simulink model "Dyn_6DoF_v2_0_r2019b"  (R2019b)
settings: Solver=ode4  StartTime=0.0  StopTime=simInit.TSIM  FixedStep=simInit.dt  MaxStep=simInit.dt  RelTol=1e-3
InitFcn:
  | close all
undefined symbols (not defined in the file): __PRM__SERIALIZED__DATA__, act, constr, DE2019, DiscIntNeverNeededParam, ENVMT, omega_rate_max, params, simInit, SubsystemReferenceBlock
libraries: simulink x16, simulink_extras x3
(part 1 of 3)
Description:
  | % Copyright 2020 Delft University of Technology
  | %
  | % Licensed under the Apache License, Version 2.0 (the "License");
  | % you may not use this file except in compliance with the License.
  | % You may obtain a copy of the License at
  | %
  | %      http://www.apache.org/licenses/LICENSE-2.0
  | %
  | % Unless required by applicable law or agreed to in writing, software
  | % distributed under the License is distributed on an "AS IS" BASIS,
  | % WITHOUT WARRANTIES OR CONDITIONS OF ANY KIND, either express or implied.
  | % See the License for the specific language governing permissions and
  | % limitations under the License.
settings Model: SimulationMode=accelerator  NumberOfSteps=50  ExtModeTrigDuration=100  Creator=Sebastian  LastModifiedBy=dylaneijkelhof
settings SolverCC: SolverJacobianMethodControl=FullAnalytical
settings DataIOCC: InitialState=testPoint  SaveFormat=Structure  SignalLogging=off  DSMLogging=off  SaveTime=off  ReturnWorkspaceOutputs=off  StateSaveName=tmp_raccel_xout  SignalLoggingName=logged_signals  LoggingFileName=log
settings OptimizationCC: BlockReduction=off  EfficientMapNaN2IntZero=off  LifeSpan=inf
settings DebuggingCC: ArtificialAlgebraicLoopMsg=none  SaveWithDisabledLinksMsg=none  SaveWithParameterizedLinksMsg=none  MaskedZcDiagnostic=none  IgnoredZcDiagnostic=none  InheritedTsInSrcMsg=none  TasksWithSamePriorityMsg=none  SigSpecEnsureSampleTimeMsg=none  ParameterPrecisionLossMsg=none  UnconnectedInputMsg=none  UnconnectedOutputMsg=none  UnconnectedLineMsg=none  BusObjectLabelMismatch=none  RootOutportRequireBusObject=none  UnknownTsInhSupMsg=none  ModelReferenceDataLoggingMessage=none  ModelReferenceSymbolNameMessage=none  InitInArrayFormatMsg=none  SFUnusedDataAndEventsDiag=none  SFUnexpectedBacktrackingDiag=none  SFInvalidInputDataAccessInChartInitDiag=none  SFNoUnconditionalDefaultTransitionDiag=none  SFTransitionOutsideNaturalParentDiag=none  SFUnreachableExecutionPathDiag=none  SFUndirectedBroadcastEventsDiag=none  SFTransitionActionBeforeConditionDiag=none  SFTemporalDelaySmallerThanSampleTimeDiag=none  SFSelfTransitionDiag=none  SFExecutionAtInitializationDiag=none  SFMachineParentedDataDiag=none  UnitsInconsistencyMsg=none  ArithmeticOperatorsInVariantConditions=warning
settings HardwareCC: ProdBitPerLong=64  ProdLongLongMode=on  ProdHWDeviceType=Custom Processor->Custom Processor  TargetBitPerLong=64  TargetBitPerPointer=64  TargetBitPerSizeT=64  TargetBitPerPtrDiffT=64  TargetLargestAtomicFloat=Float  TargetLongLongMode=on  TargetIntDivRoundTo=Zero  TargetEndianess=LittleEndian  TargetWordSize=64  TargetHWDeviceType=Custom Processor->MATLAB Host Computer
settings ModelReferenceCC: PropagateSignalLabelsOutOfModel=off
settings SFSimCC: SimUseLocalCustomCode=off  CustomCodeUndefinedFunction=UseInterfaceOnly
settings CodeAppCC: MaxIdLength=128
settings GRTTargetCC: TargetLangStandard=C89/C90 (ANSI)  CombineOutputUpdateFcns=off  GRTInterface=on
settings ConfigComp: CovMetricSettings=dw  CovHtmlReporting=on  CovSaveCumulativeToWorkspaceVar=on  CovSaveSingleToWorkspaceVar=on  CovExternalEMLEnable=off
settings SimscapeCC: SimscapeNormalizeSystem=off
settings ConfigurationSet: Description=SimMechanics 2G

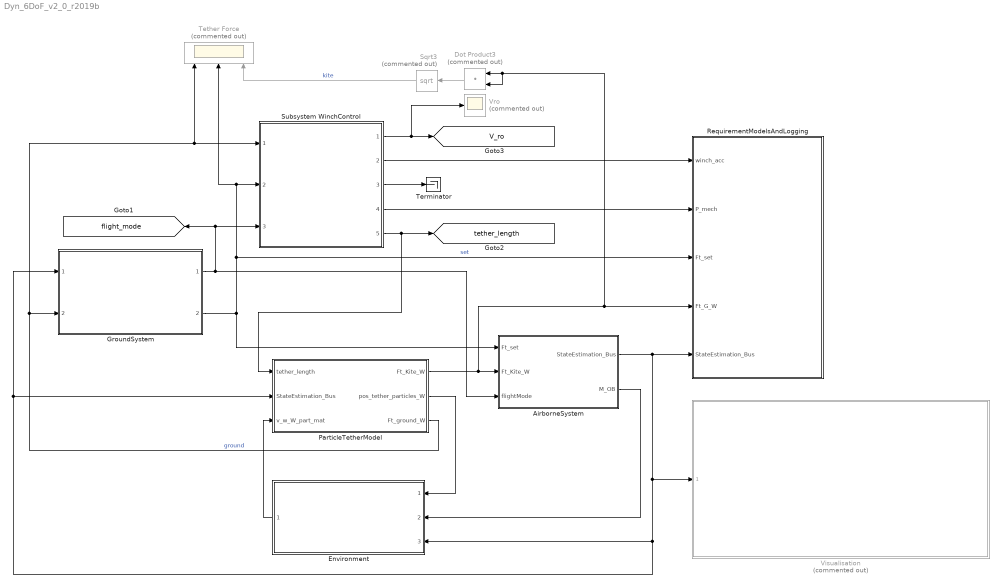
== system Dyn_6DoF_v2_0_r2019b ==
  AirborneSystem : Subsystem
  Dot Product3 : DotProduct  Commented=on  InputSameDT=on  OutDataTypeStr=Inherit: Inherit via internal rule
  Environment : Subsystem  BlockKeywords=__PRM__SERIALIZED__DATA__:SubsystemReferenceBlock  ReferencedSubsystem=Environment
  GroundSystem : Subsystem  BlockKeywords=__PRM__SERIALIZED__DATA__:SubsystemReferenceBlock  ReferencedSubsystem=GroundSystem
  ParticleTetherModel : Subsystem
  RequirementModelsAndLogging : Subsystem  mask{log_sample_time=0.2}
  Sqrt3 : Sqrt  Commented=on  SaturateOnIntegerOverflow=on
  Subsystem WinchControl : Subsystem  BlockKeywords=__PRM__SERIALIZED__DATA__:SubsystemReferenceBlock  ReferencedSubsystem=WinchControl
  Terminator : Terminator
  Tether Force : Scope  Commented=on  NumInputPorts=3
  Visualisation : Subsystem  Commented=on  ReferencedSubsystem=Visualisation
  Vro : Scope  Commented=on
  tag scope: V_ro=global, flight_mode=global, tether_length=global
  wires:
  GroundSystem/1 -> AirborneSystem/3(flightMode), Subsystem WinchControl/3, [flight_mode]
  GroundSystem/2 -> Subsystem WinchControl/2, Tether Force/2, RequirementModelsAndLogging/3(Ft_set), AirborneSystem/1(Ft_set)  "set"
  AirborneSystem/2(M_OB) -> Environment/2
  AirborneSystem/1(StateEstimation_Bus) -> RequirementModelsAndLogging/5(StateEstimation_Bus), Environment/3, GroundSystem/1, ParticleTetherModel/2(StateEstimation_Bus), Visualisation/1
  ParticleTetherModel/2(pos_tether_particles_W) -> Environment/1
  Environment/1 -> ParticleTetherModel/3(v_w_W_part_mat)
  Subsystem WinchControl/1 -> Vro/1, [V_ro]
  ParticleTetherModel/3(Ft_ground_W) -> GroundSystem/2, Subsystem WinchControl/1, Tether Force/1  "ground"
  Subsystem WinchControl/3 -> Terminator/1
  Subsystem WinchControl/2 -> RequirementModelsAndLogging/1(winch_acc)
  Subsystem WinchControl/4 -> RequirementModelsAndLogging/2(P_mech)
  Subsystem WinchControl/5 -> [tether_length], ParticleTetherModel/1(tether_length)
  Sqrt3/1 -> Tether Force/3  "kite"
  Dot Product3/1 -> Sqrt3/1
  ParticleTetherModel/1(Ft_Kite_W) -> RequirementModelsAndLogging/4(Ft_G_W), Dot Product3/2, Dot Product3/1, AirborneSystem/2(Ft_Kite_W)

== system Dyn_6DoF_v2_0_r2019b/AirborneSystem ==
  Ft_set : Inport
  Ft_Kite_W : Inport  Port=2
  flightMode : Inport  Port=3
  6DoFDynamics : Subsystem
  Dot Product : DotProduct  InputSameDT=on  OutDataTypeStr=Inherit: Inherit via internal rule
  FlightControlSystem : Subsystem
  ForcesAndTorques : Subsystem
  Sqrt : Sqrt  SaturateOnIntegerOverflow=on
  StateEstimation_Bus : Outport  VectorParamsAs1DForOutWhenUnconnected=off
  M_OB : Outport  Port=2  VectorParamsAs1DForOutWhenUnconnected=off
  wires:
  6DoFDynamics/2(StateEstimation_Bus) -> FlightControlSystem/4(StateEstimation_Bus), ForcesAndTorques/3(StateEstimation_Bus), StateEstimation_Bus/1  "StateEstimation_Bus"
  6DoFDynamics/1(M_OB) -> M_OB/1
  Ft_Kite_W/1 -> 6DoFDynamics/1(F_t_W), Dot Product/2, Dot Product/1
  Dot Product/1 -> Sqrt/1
  Ft_set/1 -> FlightControlSystem/2(Ft_set)
  Sqrt/1 -> FlightControlSystem/3(Ft_tot_kite)
  ForcesAndTorques/1(F_a_B) -> 6DoFDynamics/2(F_a_B), FlightControlSystem/1(F_a_B)
  FlightControlSystem/2(throttle/brake) -> ForcesAndTorques/2(throttle/brake)
  ForcesAndTorques/2(F_p_B) -> 6DoFDynamics/3(F_p_B)
  ForcesAndTorques/3(M_a_B) -> 6DoFDynamics/4(Torques), FlightControlSystem/5(M_a_B)
  FlightControlSystem/1(u_controlsurfaces) -> ForcesAndTorques/1(u_cmd)
  flightMode/1 -> FlightControlSystem/6(fm)

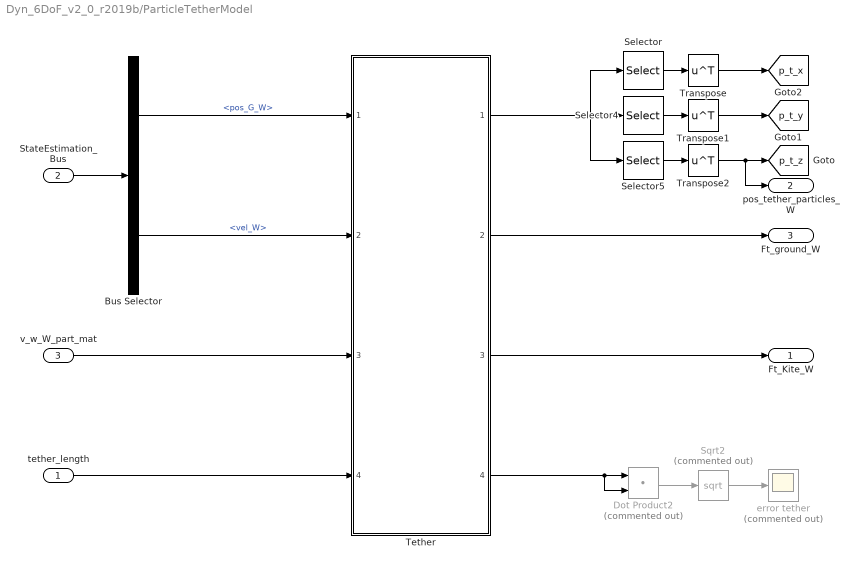
== system Dyn_6DoF_v2_0_r2019b/ParticleTetherModel ==
  tether_length : Inport
  StateEstimation_Bus : Inport  Port=2
  v_w_W_part_mat : Inport  Port=3
  Bus Selector : BusSelector  OutputSignals=pos_G_W,vel_W
  Dot Product2 : DotProduct  Commented=on  InputSameDT=on  OutDataTypeStr=Inherit: Inherit via internal rule
  Selector : Selector  NumberOfDimensions=2  InputPortWidth=3  IndexOptions=Index vector (dialog),Select all  Indices=1,1  OutputSizes=1,1
  Selector4 : Selector  NumberOfDimensions=2  InputPortWidth=3  IndexOptions=Index vector (dialog),Select all  Indices=2,1  OutputSizes=1,1
  Selector5 : Selector  NumberOfDimensions=2  InputPortWidth=3  IndexOptions=Index vector (dialog),Select all  Indices=3,1  OutputSizes=1,1
  Sqrt2 : Sqrt  Commented=on  SaturateOnIntegerOverflow=on
  Tether : Subsystem  ReferencedSubsystem=Tether_dynamics_R2019B
  Transpose : Math  Operator=transpose  SignedPower=off  SaturateOnIntegerOverflow=on
  Transpose1 : Math  Operator=transpose  SignedPower=off  SaturateOnIntegerOverflow=on
  Transpose2 : Math  Operator=transpose  SignedPower=off  SaturateOnIntegerOverflow=on
  error tether : Scope  Commented=on
  Ft_Kite_W : Outport  VectorParamsAs1DForOutWhenUnconnected=off
  pos_tether_particles_W : Outport  Port=2  VectorParamsAs1DForOutWhenUnconnected=off
  Ft_ground_W : Outport  Port=3  VectorParamsAs1DForOutWhenUnconnected=off
  tag scope: p_t_x=global, p_t_y=global, p_t_z=global
  wires:
  v_w_W_part_mat/1 -> Tether/3
  StateEstimation_Bus/1 -> Bus Selector/1
  Bus Selector/1 -> Tether/1  "<pos_G_W>"
  Bus Selector/2 -> Tether/2  "<vel_W>"
  Selector4/1 -> Transpose1/1
  Selector5/1 -> Transpose2/1
  Selector/1 -> Transpose/1
  Transpose/1 -> [p_t_x]
  Transpose1/1 -> [p_t_y]
  Transpose2/1 -> pos_tether_particles_W/1, [p_t_z]
  Tether/4 -> Dot Product2/2, Dot Product2/1
  Tether/1 -> Selector/1, Selector5/1, Selector4/1
  Dot Product2/1 -> Sqrt2/1
  Sqrt2/1 -> error tether/1
  Tether/2 -> Ft_ground_W/1
  Tether/3 -> Ft_Kite_W/1
  tether_length/1 -> Tether/4

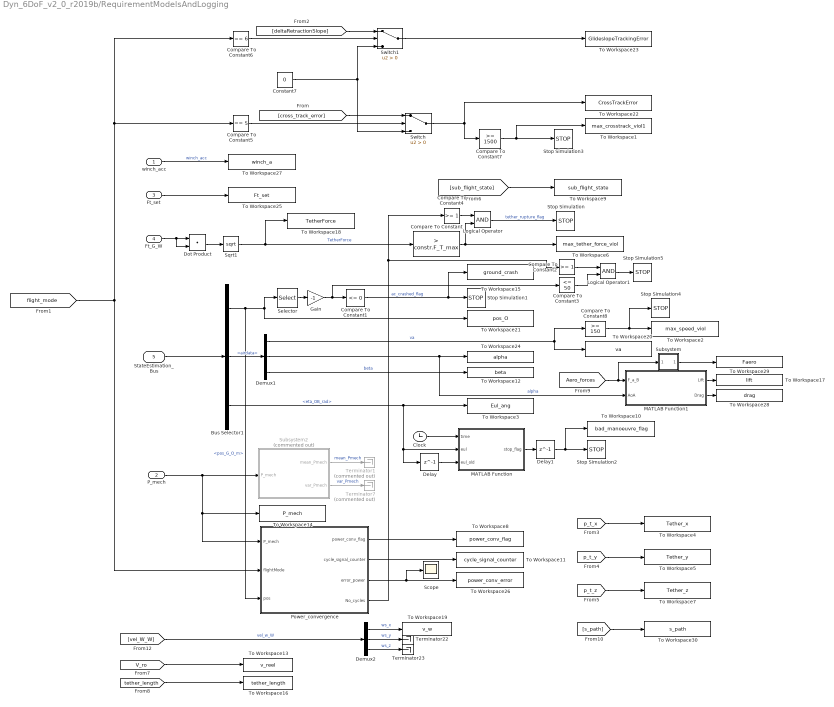
== system Dyn_6DoF_v2_0_r2019b/RequirementModelsAndLogging ==
  winch_acc : Inport
  P_mech : Inport  Port=2
  Ft_set : Inport  Port=3
  Ft_G_W : Inport  Port=4
  StateEstimation_Bus : Inport  Port=5
  Bus Selector1 : BusSelector  OutputSignals=pos_G_O_m,airdata,eta_OB_rad
  Clock : Clock
  Compare To Constant : simulink/Logic and Bit Operations/Compare To Constant  relop=>  const=constr.F_T_max  OutDataTypeStr=boolean
  Compare To Constant1 : simulink/Logic and Bit Operations/Compare To Constant  relop=<=  const=0  OutDataTypeStr=boolean
  Compare To Constant2 : simulink/Logic and Bit Operations/Compare To Constant  relop=>=  const=1  OutDataTypeStr=boolean
  Compare To Constant3 : simulink/Logic and Bit Operations/Compare To Constant  relop=<=  const=50  OutDataTypeStr=boolean
  Compare To Constant4 : simulink/Logic and Bit Operations/Compare To Constant  relop=>=  const=1  OutDataTypeStr=boolean
  Compare To Constant5 : simulink/Logic and Bit Operations/Compare To Constant  relop===  const=5  OutDataTypeStr=boolean
  Compare To Constant6 : simulink/Logic and Bit Operations/Compare To Constant  relop===  const=6  OutDataTypeStr=boolean
  Compare To Constant7 : simulink/Logic and Bit Operations/Compare To Constant  relop=>=  const=1500  OutDataTypeStr=boolean
  Compare To Constant8 : simulink/Logic and Bit Operations/Compare To Constant  relop=>=  const=150  OutDataTypeStr=boolean
  Constant7 : Constant  Value=0
  Delay : Delay  DelayLength=1  InitialCondition=zeros(3,1)
  Delay1 : Delay  DelayLength=1
  Demux1 : Demux  Outputs=3
  Demux2 : Demux  Outputs=3
  Dot Product : DotProduct  InputSameDT=on  OutDataTypeStr=Inherit: Inherit via internal rule
  Gain : Gain  Gain=-1
  Logical Operator : Logic  AllPortsSameDT=off  OutDataTypeStr=boolean
  Logical Operator1 : Logic  AllPortsSameDT=off  OutDataTypeStr=boolean
  MATLAB Function : MATLAB Function  TreatAsAtomicUnit=on
  MATLAB Function1 : MATLAB Function  TreatAsAtomicUnit=on
  Power_convergence : Subsystem  mask{sample_time=simInit.Ts_power_conv_check, threshold=130000, min_cycles=3, pos_threshold=400}
      mask prompts: threshold "start_threshold"; min_cycles "minimum_cycles"; pos_threshold "maximum position distance"
  Scope : Scope
  Selector : Selector  InputPortWidth=3  IndexOptions=Index vector (dialog)  Indices=3  OutputSizes=1
  Sqrt1 : Sqrt  SaturateOnIntegerOverflow=on
  Stop Simulation{,1..5} (6 alike) : Stop
  Subsystem : Subsystem
      mask Display: disp('norm()')
  Subsystem2 : Subsystem  Commented=on
  Switch : Switch  Criteria=u2 > Threshold
  Switch1 : Switch  Criteria=u2 > Threshold
  Terminator1 : Terminator  Commented=on
  Terminator22 : Terminator
  Terminator23 : Terminator
  Terminator7 : Terminator  Commented=on
  To Workspace1 : ToWorkspace  VariableName=max_crosstrack_viol1  SampleTime=-1
      settings: MaxDataPoints=1
  To Workspace10 : ToWorkspace  VariableName=bad_manoeuvre_flag  SampleTime=-1
      settings: MaxDataPoints=1
  To Workspace11 : ToWorkspace  VariableName=cycle_signal_counter  SaveFormat=Timeseries  SampleTime=-1
      settings: MaxDataPoints=1  Save2DSignal=2-D array (concatenate along first dimension)
  To Workspace12 : ToWorkspace  VariableName=beta  SaveFormat=Timeseries  SampleTime=simInit.AttLoggingTs
      settings: Save2DSignal=2-D array (concatenate along first dimension)
  To Workspace13 : ToWorkspace  VariableName=v_reel  SaveFormat=Timeseries  SampleTime=simInit.PLoggingTs
  To Workspace14 : ToWorkspace  VariableName=P_mech  SaveFormat=Timeseries  SampleTime=simInit.PLoggingTs
  To Workspace15 : ToWorkspace  VariableName=ground_crash  SampleTime=-1
      settings: MaxDataPoints=1
  To Workspace16 : ToWorkspace  VariableName=tether_length  SaveFormat=Timeseries  SampleTime=simInit.AttLoggingTs
  To Workspace17 : ToWorkspace  VariableName=lift  SaveFormat=Timeseries  SampleTime=simInit.AttLoggingTs
      settings: Save2DSignal=2-D array (concatenate along first dimension)
  To Workspace18 : ToWorkspace  VariableName=TetherForce  SaveFormat=Timeseries  SampleTime=simInit.FtLoggingTs
  To Workspace19 : ToWorkspace  VariableName=v_w  SaveFormat=Timeseries  SampleTime=simInit.PLoggingTs
  To Workspace2 : ToWorkspace  VariableName=max_speed_viol  SampleTime=-1
      settings: MaxDataPoints=1
  To Workspace20 : ToWorkspace  VariableName=va  SaveFormat=Timeseries  SampleTime=simInit.AttLoggingTs
      settings: Save2DSignal=2-D array (concatenate along first dimension)
  To Workspace21 : ToWorkspace  VariableName=pos_O  SaveFormat=Timeseries  SampleTime=simInit.PLoggingTs
      settings: Save2DSignal=2-D array (concatenate along first dimension)
  To Workspace22 : ToWorkspace  VariableName=CrossTrackError  SaveFormat=Timeseries  SampleTime=simInit.CteLoggingTs
      settings: Save2DSignal=2-D array (concatenate along first dimension)
  To Workspace23 : ToWorkspace  VariableName=GlideslopeTrackingError  SaveFormat=Timeseries  SampleTime=simInit.GSLoggingTs
      settings: Save2DSignal=2-D array (concatenate along first dimension)
  To Workspace24 : ToWorkspace  VariableName=alpha  SaveFormat=Timeseries  SampleTime=simInit.AttLoggingTs
      settings: Save2DSignal=2-D array (concatenate along first dimension)
  To Workspace25 : ToWorkspace  VariableName=Ft_set  SaveFormat=Timeseries  SampleTime=simInit.FtLoggingTs
  To Workspace26 : ToWorkspace  VariableName=power_conv_error  SaveFormat=Timeseries  SampleTime=-1
      settings: Save2DSignal=2-D array (concatenate along first dimension)
  To Workspace27 : ToWorkspace  VariableName=winch_a  SaveFormat=Timeseries  SampleTime=simInit.PLoggingTs
  To Workspace28 : ToWorkspace  VariableName=drag  SaveFormat=Timeseries  SampleTime=simInit.AttLoggingTs
      settings: Save2DSignal=2-D array (concatenate along first dimension)
  To Workspace29 : ToWorkspace  VariableName=Faero  SaveFormat=Timeseries  SampleTime=simInit.AttLoggingTs
      settings: Save2DSignal=2-D array (concatenate along first dimension)
  To Workspace3 : ToWorkspace  VariableName=Eul_ang  SaveFormat=Timeseries  SampleTime=simInit.PLoggingTs
      settings: Save2DSignal=2-D array (concatenate along first dimension)
  To Workspace30 : ToWorkspace  VariableName=s_path  SaveFormat=Timeseries  SampleTime=simInit.PLoggingTs
      settings: Save2DSignal=2-D array (concatenate along first dimension)
  To Workspace4 : ToWorkspace  VariableName=Tether_x  SaveFormat=Timeseries  SampleTime=simInit.PLoggingTs
      settings: Save2DSignal=2-D array (concatenate along first dimension)
  To Workspace5 : ToWorkspace  VariableName=Tether_y  SaveFormat=Timeseries  SampleTime=simInit.PLoggingTs
      settings: Save2DSignal=2-D array (concatenate along first dimension)
  To Workspace6 : ToWorkspace  VariableName=max_tether_force_viol  SampleTime=-1
      settings: MaxDataPoints=1
  To Workspace7 : ToWorkspace  VariableName=Tether_z  SaveFormat=Timeseries  SampleTime=simInit.PLoggingTs
      settings: Save2DSignal=2-D array (concatenate along first dimension)
  To Workspace8 : ToWorkspace  VariableName=power_conv_flag  SampleTime=-1
      settings: MaxDataPoints=1
  To Workspace9 : ToWorkspace  VariableName=sub_flight_state  SaveFormat=Timeseries  SampleTime=simInit.FtLoggingTs
  wires:
  Bus Selector1/1 -> Power_convergence/3(pos), Selector/1, To Workspace21/1  "<pos_G_O_m>"
  Gain/1 -> Compare To Constant3/1, Compare To Constant1/1
  Compare To Constant1/1 -> To Workspace15/1, Stop Simulation1/1  "ac_crashed_flag"
  Selector/1 -> Gain/1
  winch_acc/1 -> To Workspace27/1  "winch_acc"
  Logical Operator/1 -> Stop Simulation/1  "tether_rupture_flag"
  Sqrt1/1 -> To Workspace18/1, Compare To Constant/1  "TetherForce"
  StateEstimation_Bus/1 -> Bus Selector1/1
  Power_convergence/1(power_conv_flag) -> To Workspace8/1
  Power_convergence/2(cycle_signal_counter) -> To Workspace11/1
  [vel_W_W] -> Demux2/1  "vel_w_W"
  Bus Selector1/2 -> Demux1/1  "<airdata>"
  Switch/1 -> To Workspace22/1, Compare To Constant7/1
  Subsystem2/1(mean_Pmech) -> Terminator1/1  "mean_Pmech"
  Subsystem2/2(var_Pmech) -> Terminator7/1  "var_Pmech"
  Demux1/1 -> To Workspace20/1, Compare To Constant8/1  "va"
  Demux1/2 -> MATLAB Function1/2(AoA), To Workspace24/1  "alpha"
  Demux1/3 -> To Workspace12/1  "beta"
  Demux2/3 -> Terminator23/1  "ws_z"
  Demux2/2 -> Terminator22/1  "ws_y"
  Demux2/1 -> To Workspace19/1  "ws_x"
  Ft_G_W/1 -> Dot Product/2, Dot Product/1
  Dot Product/1 -> Sqrt1/1
  Clock/1 -> MATLAB Function/1(time)
  Compare To Constant4/1 -> Logical Operator/1
  Compare To Constant/1 -> Logical Operator/2, To Workspace6/1
  [flight_mode] -> Compare To Constant6/1, Compare To Constant5/1, Power_convergence/2(flightMode)
  P_mech/1 -> Power_convergence/1(P_mech), To Workspace14/1, Subsystem2/1(P_mech)
  Compare To Constant5/1 -> Switch/2
  [cross_track_error] -> Switch/1
  Switch1/1 -> To Workspace23/1
  [deltaRetractionSlope] -> Switch1/1
  Compare To Constant6/1 -> Switch1/2
  Constant7/1 -> Switch1/3, Switch/3
  Ft_set/1 -> To Workspace25/1
  Power_convergence/3(error_power) -> Scope/1, To Workspace26/1
  Compare To Constant7/1 -> Stop Simulation3/1, To Workspace1/1
  Compare To Constant8/1 -> To Workspace2/1, Stop Simulation4/1
  Bus Selector1/3 -> Delay/1, MATLAB Function/2(eul), To Workspace3/1  "<eta_OB_rad>"
  [p_t_y] -> To Workspace5/1
  [p_t_x] -> To Workspace4/1
  [p_t_z] -> To Workspace7/1
  [sub_flight_state] -> To Workspace9/1
  Delay/1 -> MATLAB Function/3(eul_old)
  MATLAB Function/1(stop_flag) -> Delay1/1
  Delay1/1 -> Stop Simulation2/1, To Workspace10/1
  [V_ro] -> To Workspace13/1
  [tether_length] -> To Workspace16/1
  [Aero_forces] -> Subsystem/1(In1), MATLAB Function1/1(F_a_B)
  MATLAB Function1/1(Lift) -> To Workspace17/1
  MATLAB Function1/2(Drag) -> To Workspace28/1
  Power_convergence/4(No_cycles) -> Compare To Constant2/1, Compare To Constant4/1
  Compare To Constant2/1 -> Logical Operator1/1
  Compare To Constant3/1 -> Logical Operator1/2
  Logical Operator1/1 -> Stop Simulation5/1
  Subsystem/1(Out1) -> To Workspace29/1
  [s_path] -> To Workspace30/1

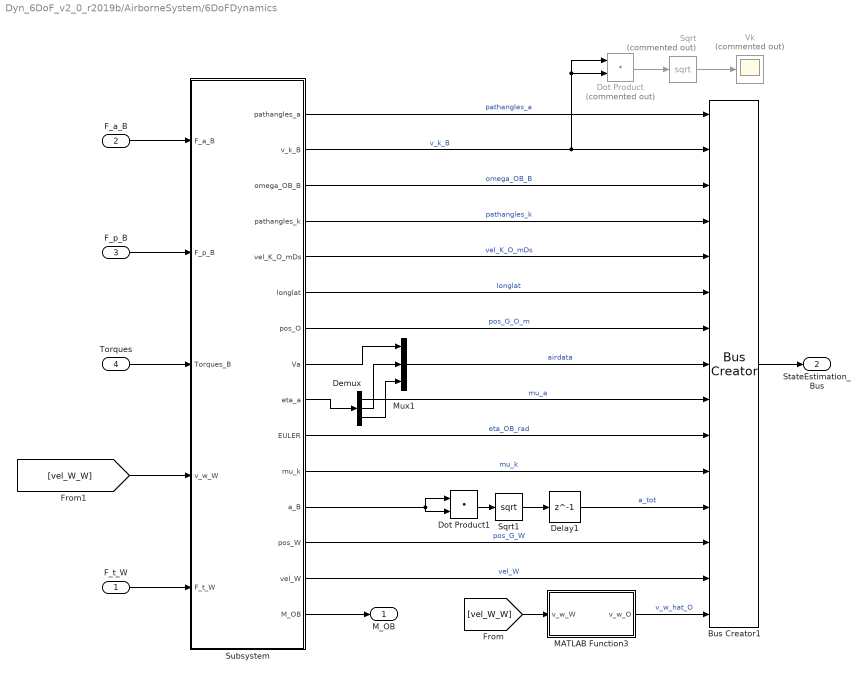
== system Dyn_6DoF_v2_0_r2019b/AirborneSystem/6DoFDynamics ==
  F_t_W : Inport
  F_a_B : Inport  Port=2
  F_p_B : Inport  Port=3
  Torques : Inport  Port=4
  Bus Creator1 : BusCreator  Inputs=15
  Delay1 : Delay  DelayLength=1
  Demux : Demux  Outputs=3
  Dot Product : DotProduct  Commented=on  InputSameDT=on  OutDataTypeStr=Inherit: Inherit via internal rule
  Dot Product1 : DotProduct  InputSameDT=on  OutDataTypeStr=Inherit: Inherit via internal rule
  MATLAB Function3 : MATLAB Function  TreatAsAtomicUnit=on
  Mux1 : Mux  Inputs=3
  Sqrt : Sqrt  Commented=on  SaturateOnIntegerOverflow=on
  Sqrt1 : Sqrt  SaturateOnIntegerOverflow=on
  Subsystem : Subsystem
  Vk : Scope  Commented=on
  M_OB : Outport  PortDimensions=[3,3]  VectorParamsAs1DForOutWhenUnconnected=off
  StateEstimation_Bus : Outport  Port=2  VectorParamsAs1DForOutWhenUnconnected=off
  wires:
  Demux/1 -> Bus Creator1/9  "mu_a"
  Subsystem/15(M_OB) -> M_OB/1
  Subsystem/8(Va) -> Mux1/1
  Subsystem/1(pathangles_a) -> Bus Creator1/1  "pathangles_a"
  [vel_W_W] -> Subsystem/4(v_w_W)
  Torques/1 -> Subsystem/3(Torques_B)
  F_p_B/1 -> Subsystem/2(F_p_B)
  F_a_B/1 -> Subsystem/1(F_a_B)
  Subsystem/4(pathangles_k) -> Bus Creator1/4  "pathangles_k"
  Subsystem/2(v_k_B) -> Bus Creator1/2, Dot Product/1, Dot Product/2  "v_k_B"
  Subsystem/10(EULER) -> Bus Creator1/10  "eta_OB_rad"
  Subsystem/6(longlat) -> Bus Creator1/6  "longlat"
  Subsystem/5(vel_K_O_mDs) -> Bus Creator1/5  "vel_K_O_mDs"
  Bus Creator1/1 -> StateEstimation_Bus/1
  Subsystem/3(omega_OB_B) -> Bus Creator1/3  "omega_OB_B"
  Subsystem/7(pos_O) -> Bus Creator1/7  "pos_G_O_m"
  Demux/3 -> Mux1/3
  Subsystem/9(eta_a) -> Demux/1
  Delay1/1 -> Bus Creator1/12  "a_tot"
  Sqrt1/1 -> Delay1/1
  Dot Product1/1 -> Sqrt1/1
  Subsystem/12(a_B) -> Dot Product1/1, Dot Product1/2
  Subsystem/11(mu_k) -> Bus Creator1/11  "mu_k"
  MATLAB Function3/1(v_w_O) -> Bus Creator1/15  "v_w_hat_O"
  [vel_W_W] -> MATLAB Function3/1(v_w_W)
  Mux1/1 -> Bus Creator1/8  "airdata"
  Demux/2 -> Mux1/2
  F_t_W/1 -> Subsystem/5(F_t_W)
  Subsystem/13(pos_W) -> Bus Creator1/13  "pos_G_W"
  Subsystem/14(vel_W) -> Bus Creator1/14  "vel_W"
  Sqrt/1 -> Vk/1
  Dot Product/1 -> Sqrt/1

== system Dyn_6DoF_v2_0_r2019b/AirborneSystem/FlightControlSystem ==
  F_a_B : Inport
  Ft_set : Inport  Port=2
  Ft_tot_kite : Inport  Port=3
  StateEstimation_Bus : Inport  Port=4
  M_a_B : Inport  Port=5
  fm : Inport  Port=6
  AirspeedController : Subsystem  BlockKeywords=__PRM__SERIALIZED__DATA__:SubsystemReferenceBlock  ReferencedSubsystem=AirspeedController
  AoA : Scope  NumInputPorts=2
  AttitudeAndRateLoop : Subsystem
  Bus Selector : BusSelector  OutputSignals=airdata,pathangles_a,v_k_B
  PathFollowingController : Subsystem  BlockKeywords=__PRM__SERIALIZED__DATA__:SubsystemReferenceBlock  ReferencedSubsystem=PathFollowingController
  Selector : Selector  InputPortWidth=3  IndexOptions=Index vector (dialog)  Indices=1  OutputSizes=1
  Selector1 : Selector  InputPortWidth=3  IndexOptions=Index vector (dialog)  Indices=2  OutputSizes=1
  Selector2 : Selector  InputPortWidth=2  IndexOptions=Index vector (dialog)  Indices=2  OutputSizes=1
  Va : Scope
  u_controlsurfaces : Outport  VectorParamsAs1DForOutWhenUnconnected=off
  throttle/brake : Outport  Port=2  VectorParamsAs1DForOutWhenUnconnected=off
  wires:
  StateEstimation_Bus/1 -> PathFollowingController/4, Bus Selector/1, AttitudeAndRateLoop/5(StateEstimation_Bus)
  Ft_set/1 -> PathFollowingController/1
  Ft_tot_kite/1 -> AirspeedController/6, PathFollowingController/2
  Bus Selector/1 -> Selector/1, Selector1/1  "<airdata>"
  Selector2/1 -> AirspeedController/3
  Selector/1 -> AirspeedController/1, Va/1
  Selector1/1 -> AirspeedController/2, AoA/1
  F_a_B/1 -> AirspeedController/5, PathFollowingController/3
  Bus Selector/2 -> Selector2/1  "<pathangles_a>"
  AirspeedController/1 -> throttle/brake/1
  AttitudeAndRateLoop/1(u_rb) -> u_controlsurfaces/1
  PathFollowingController/1 -> AttitudeAndRateLoop/1(mu_a_cmd)
  PathFollowingController/2 -> AttitudeAndRateLoop/4(alpha_a_cmd), AoA/2
  M_a_B/1 -> AttitudeAndRateLoop/2(M_a_B_est)
  fm/1 -> AttitudeAndRateLoop/3(flightMode)
  Bus Selector/3 -> AirspeedController/4  "<v_k_B>"

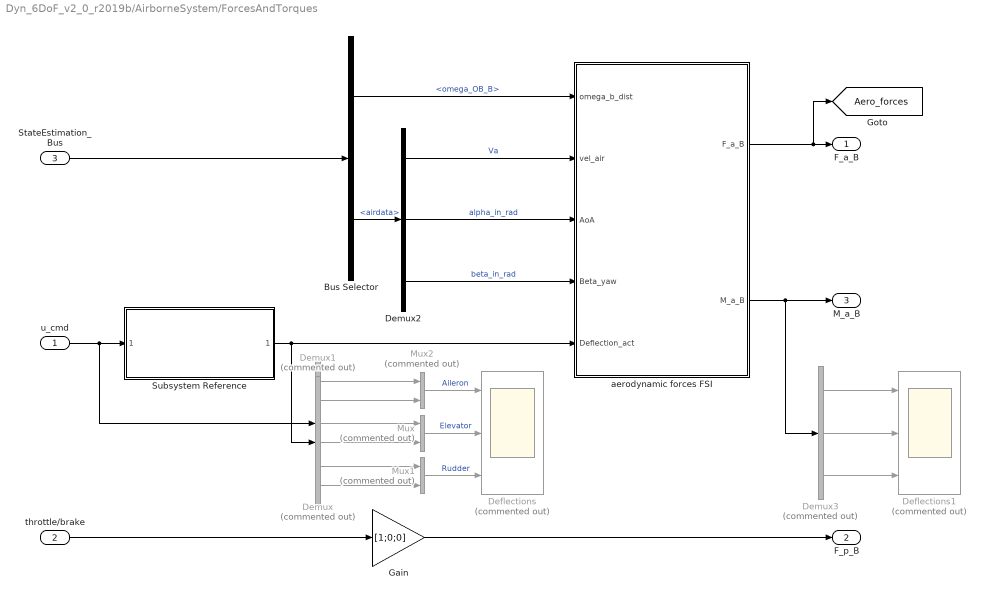
== system Dyn_6DoF_v2_0_r2019b/AirborneSystem/ForcesAndTorques ==
  u_cmd : Inport
  throttle/brake : Inport  Port=2
  StateEstimation_Bus : Inport  Port=3
  Bus Selector : BusSelector  OutputSignals=omega_OB_B,airdata
  Deflections : Scope  Commented=on  NumInputPorts=3
  Deflections1 : Scope  Commented=on  NumInputPorts=3
  Demux : Demux  Commented=on  Outputs=3
  Demux1 : Demux  Commented=on  Outputs=3
  Demux2 : Demux  Outputs=3
  Demux3 : Demux  Commented=on  Outputs=3
  Gain : Gain  Gain=[1;0;0]
  Mux : Mux  Commented=on  Inputs=2
  Mux1 : Mux  Commented=on  Inputs=2
  Mux2 : Mux  Commented=on  Inputs=2
  Subsystem Reference : Subsystem  ReferencedSubsystem=Actuatormodel_R2019B
  aerodynamic forces FSI : Subsystem
  F_a_B : Outport  VectorParamsAs1DForOutWhenUnconnected=off
  F_p_B : Outport  Port=2  VectorParamsAs1DForOutWhenUnconnected=off
  M_a_B : Outport  Port=3  VectorParamsAs1DForOutWhenUnconnected=off
  tag scope: Aero_forces=global
  wires:
  Bus Selector/2 -> Demux2/1  "<airdata>"
  StateEstimation_Bus/1 -> Bus Selector/1
  throttle/brake/1 -> Gain/1
  Gain/1 -> F_p_B/1
  u_cmd/1 -> Subsystem Reference/1, Demux/1
  Bus Selector/1 -> aerodynamic forces FSI/1(omega_b_dist)  "<omega_OB_B>"
  Subsystem Reference/1 -> aerodynamic forces FSI/5(Deflection_act), Demux1/1
  Demux2/1 -> aerodynamic forces FSI/2(vel_air)  "Va"
  Demux2/2 -> aerodynamic forces FSI/3(AoA)  "alpha_in_rad"
  Demux2/3 -> aerodynamic forces FSI/4(Beta_yaw)  "beta_in_rad"
  Demux/1 -> Mux2/1
  Demux/3 -> Mux1/1
  Demux1/1 -> Mux2/2
  Demux/2 -> Mux/1
  Mux/1 -> Deflections/2  "Elevator"
  Mux2/1 -> Deflections/1  "Aileron"
  Mux1/1 -> Deflections/3  "Rudder"
  Demux1/2 -> Mux/2
  Demux1/3 -> Mux1/2
  aerodynamic forces FSI/1(F_a_B) -> [Aero_forces], F_a_B/1
  aerodynamic forces FSI/2(M_a_B) -> Demux3/1, M_a_B/1
  Demux3/1 -> Deflections1/1
  Demux3/2 -> Deflections1/2
  Demux3/3 -> Deflections1/3

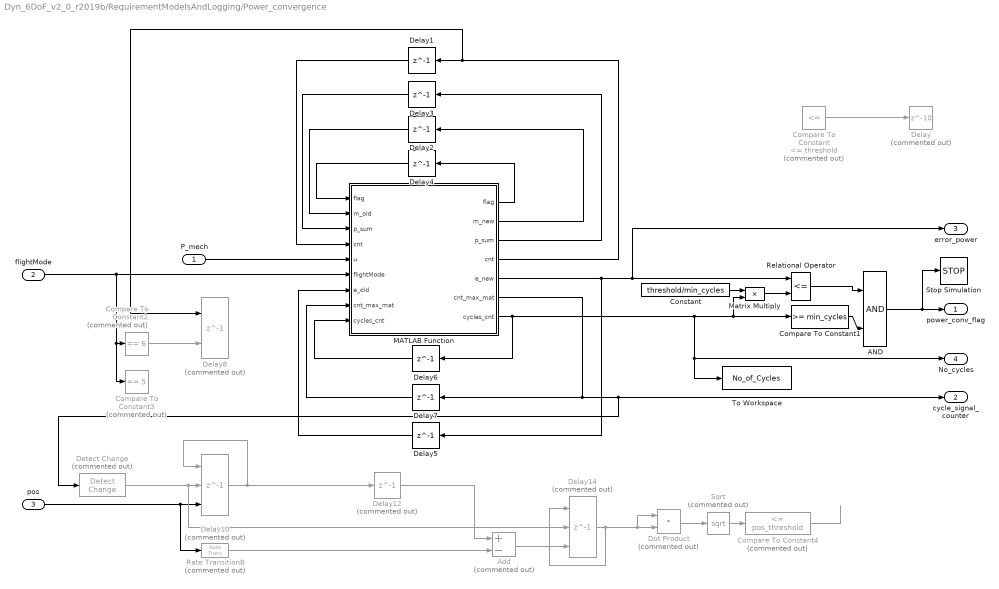
== system Dyn_6DoF_v2_0_r2019b/RequirementModelsAndLogging/Power_convergence ==
  P_mech : Inport
  flightMode : Inport  Port=2
  pos : Inport  Port=3
  AND : Logic  AllPortsSameDT=off  OutDataTypeStr=boolean
  Add : Sum  Commented=on  Inputs=+-
  Compare To Constant : simulink/Logic and Bit Operations/Compare To Constant  Commented=on  relop=<=  const=threshold  OutDataTypeStr=boolean
  Compare To Constant1 : simulink/Logic and Bit Operations/Compare To Constant  relop=>=  const=min_cycles  OutDataTypeStr=boolean
  Compare To Constant2 : simulink/Logic and Bit Operations/Compare To Constant  Commented=on  relop===  const=6  OutDataTypeStr=boolean
  Compare To Constant3 : simulink/Logic and Bit Operations/Compare To Constant  Commented=on  relop===  const=5  OutDataTypeStr=boolean
  Compare To Constant4 : simulink/Logic and Bit Operations/Compare To Constant  Commented=on  relop=<=  const=pos_threshold  OutDataTypeStr=boolean
  Constant : Constant  Value=threshold/min_cycles
  Delay : Delay  Commented=on  DelayLength=10
  Delay{1..4,6..7} (6 alike) : Delay  DelayLength=1  InitialCondition=0
  Delay10 : Delay  Commented=on  DelayLength=1  InitialConditionSource=Input port  InitialCondition=0  ExternalReset=Rising
      settings: InputPortMap=u0,r5,p4
  Delay12 : Delay  Commented=on  DelayLength=1  InitialCondition=0
  Delay14 : Delay  Commented=on  DelayLength=1  InitialConditionSource=Input port  InitialCondition=0  ExternalReset=Rising
      settings: InputPortMap=u0,r5,p4
  Delay5 : Delay  DelayLength=1  InitialCondition=threshold+1000
  Delay8 : Delay  Commented=on  DelayLength=1  InitialCondition=0  ExternalReset=Rising
      settings: InputPortMap=u0,r5
  Detect Change : simulink/Logic and Bit Operations/Detect Change  Commented=on  vinit=0  OutDataTypeStr=boolean
  Dot Product : DotProduct  Commented=on  InputSameDT=on  OutDataTypeStr=Inherit: Inherit via internal rule
  MATLAB Function : MATLAB Function  TreatAsAtomicUnit=on
  Matrix Multiply : Product
  Rate Transition8 : RateTransition  Commented=on  InitialCondition=[0;0;0]  OutPortSampleTime=sample_time
  Relational Operator : RelationalOperator  Operator=<=  OutDataTypeStr=boolean  RndMeth=Simplest
  Sqrt : Sqrt  Commented=on  SaturateOnIntegerOverflow=on
  Stop Simulation : Stop
  To Workspace : ToWorkspace  VariableName=No_of_Cycles  SaveFormat=Timeseries  SampleTime=-1
      settings: MaxDataPoints=1
  power_conv_flag : Outport  VectorParamsAs1DForOutWhenUnconnected=off
  cycle_signal_counter : Outport  Port=2  VectorParamsAs1DForOutWhenUnconnected=off
  error_power : Outport  Port=3  VectorParamsAs1DForOutWhenUnconnected=off
  No_cycles : Outport  Port=4
  wires:
  Delay1/1 -> MATLAB Function/4("cnt ")
  P_mech/1 -> MATLAB Function/5(u)
  MATLAB Function/4(cnt) -> Delay8/1, Delay1/1
  Delay2/1 -> MATLAB Function/2(m_old)
  MATLAB Function/1(flag) -> Delay4/1
  Delay4/1 -> MATLAB Function/1("flag ")
  Delay3/1 -> MATLAB Function/3("p_sum ")
  MATLAB Function/3(p_sum) -> Delay3/1
  MATLAB Function/5(e_new) -> Relational Operator/1, error_power/1, Delay5/1
  Delay5/1 -> MATLAB Function/7(e_old)
  AND/1 -> Stop Simulation/1, power_conv_flag/1
  Delay7/1 -> MATLAB Function/8("cnt_max_mat ")
  MATLAB Function/2(m_new) -> Delay2/1
  MATLAB Function/7(cycles_cnt) -> Compare To Constant1/1, Matrix Multiply/2, No_cycles/1, To Workspace/1, Delay6/1
  Delay6/1 -> MATLAB Function/9("cycles_cnt ")
  Relational Operator/1 -> AND/1
  Compare To Constant1/1 -> AND/2
  Compare To Constant2/1 -> Delay8/2
  Compare To Constant/1 -> Delay/1
  Constant/1 -> Matrix Multiply/1
  Matrix Multiply/1 -> Relational Operator/2
  pos/1 -> Rate Transition8/1, Delay10/3
  Sqrt/1 -> Compare To Constant4/1
  Dot Product/1 -> Sqrt/1
  Delay14/1 -> Delay14/1, Dot Product/1, Dot Product/2
  Rate Transition8/1 -> Add/2
  MATLAB Function/6(cnt_max_mat) -> Detect Change/1, cycle_signal_counter/1, Delay7/1
  Delay10/1 -> Delay12/1, Delay10/1
  flightMode/1 -> MATLAB Function/6(flightMode), Compare To Constant3/1, Compare To Constant2/1
  Add/1 -> Delay14/3
  Detect Change/1 -> Delay14/2, Delay10/2
  Compare To Constant4/1 -> ?
  Delay12/1 -> Add/1

== system Dyn_6DoF_v2_0_r2019b/RequirementModelsAndLogging/Subsystem ==
  In1 : Inport
  Dot Product3 : DotProduct  InputSameDT=on  OutDataTypeStr=Inherit: Inherit via internal rule
  Sqrt1 : Sqrt  SaturateOnIntegerOverflow=on
  Out1 : Outport
  wires:
  In1/1 -> Dot Product3/1, Dot Product3/2
  Sqrt1/1 -> Out1/1
  Dot Product3/1 -> Sqrt1/1

== system Dyn_6DoF_v2_0_r2019b/RequirementModelsAndLogging/Subsystem2 ==
  P_mech : Inport
  Constant7 : Constant
  Delay1 : Delay  DelayLength=1  SampleTime=0.1
  Delay3 : Delay  DelayLength=1  SampleTime=0.1
  Delay4 : Delay  DelayLength=1  InitialCondition=1  SampleTime=0.1
  Divide : Product  Inputs=*/
  Divide1 : Product  Inputs=*/
  Product : Product
  Rate Transition1 : RateTransition  OutPortSampleTime=0.1
  Rate Transition6 : RateTransition  OutPortSampleTime=0.1
  Sum : Sum  Inputs=|+-
  Sum1 : Sum  Inputs=|++
  Sum3 : Sum  Inputs=|++
  Sum4 : Sum  Inputs=|++
  To Workspace : ToWorkspace  Commented=on  VariableName=P_mech  SampleTime=log_sample_time
  mean_Pmech : Outport  VectorParamsAs1DForOutWhenUnconnected=off
  var_Pmech : Outport  Port=2  VectorParamsAs1DForOutWhenUnconnected=off
  wires:
  P_mech/1 -> Rate Transition6/1
  Delay4/1 -> Sum4/2
  Constant7/1 -> Rate Transition1/1
  Divide/1 -> mean_Pmech/1, Sum/2
  Rate Transition1/1 -> Sum4/1
  Sum3/1 -> Divide/1, Delay3/1
  Sum4/1 -> Divide1/2, Delay4/1, Divide/2
  Delay3/1 -> Sum3/2
  Sum/1 -> Product/2, Product/1
  Product/1 -> Sum1/1
  Delay1/1 -> Sum1/2
  Sum1/1 -> Divide1/1, Delay1/1
  Divide1/1 -> var_Pmech/1
  Rate Transition6/1 -> To Workspace/1, Sum/1, Sum3/1  "vel_w_W"

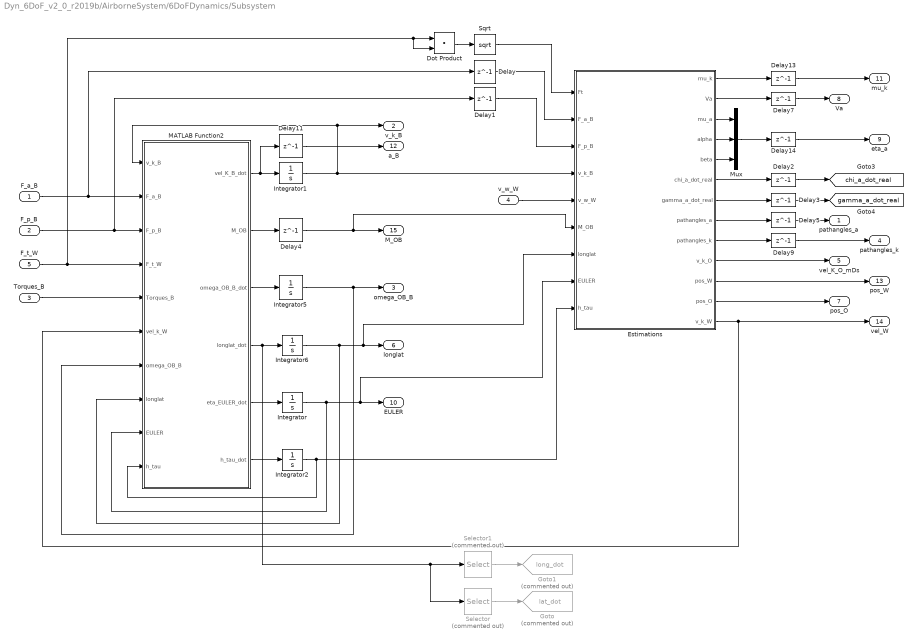
== system Dyn_6DoF_v2_0_r2019b/AirborneSystem/6DoFDynamics/Subsystem ==
  F_a_B : Inport  PortDimensions=[3,1]
  F_p_B : Inport  Port=2
  Torques_B : Inport  Port=3  PortDimensions=[3,1]
  v_w_W : Inport  Port=4  PortDimensions=[3,1]
  F_t_W : Inport  Port=5
  Delay{,1,11,14} (4 alike) : Delay  DelayLength=1  InitialCondition=zeros(3,1)
  Delay13 : Delay  DelayLength=1  InitialCondition=0
  Delay2 : Delay  DelayLength=1
  Delay3 : Delay  DelayLength=1
  Delay4 : Delay  DelayLength=1  InitialCondition=eye(3)
  Delay5 : Delay  DelayLength=1  InitialCondition=zeros(2,1)
  Delay7 : Delay  DelayLength=1  InitialCondition=simInit.vel_B_init(1)
  Delay9 : Delay  DelayLength=1  InitialCondition=zeros(2,1)
  Dot Product : DotProduct  InputSameDT=on  OutDataTypeStr=Inherit: Inherit via internal rule
  Estimations : MATLAB Function  TreatAsAtomicUnit=on
  Goto : Goto  Commented=on  GotoTag=lat_dot  TagVisibility=global
  Goto1 : Goto  Commented=on  GotoTag=long_dot  TagVisibility=global
  Integrator : Integrator  InitialCondition=simInit.eta_init  WrapState=on
  Integrator1 : Integrator  InitialCondition=simInit.vel_B_init
  Integrator2 : Integrator  InitialCondition=norm(simInit.pos_O_init)
  Integrator5 : Integrator  InitialCondition=zeros(3,1)
  Integrator6 : Integrator  InitialCondition=[simInit.long_init;simInit.lat_init]  WrapState=on
  MATLAB Function2 : MATLAB Function  TreatAsAtomicUnit=on
  Mux : Mux  Inputs=3
  Selector : Selector  Commented=on  InputPortWidth=2  IndexOptions=Index vector (dialog)  Indices=2  OutputSizes=1
  Selector1 : Selector  Commented=on  InputPortWidth=2  IndexOptions=Index vector (dialog)  Indices=1  OutputSizes=1
  Sqrt : Sqrt  SaturateOnIntegerOverflow=on
  pathangles_a : Outport  PortDimensions=[2,1]  VectorParamsAs1DForOutWhenUnconnected=off
  v_k_B : Outport  Port=2  PortDimensions=[3,1]  VectorParamsAs1DForOutWhenUnconnected=off
  omega_OB_B : Outport  Port=3  PortDimensions=[3,1]  VectorParamsAs1DForOutWhenUnconnected=off
  pathangles_k : Outport  Port=4  PortDimensions=[2,1]  VectorParamsAs1DForOutWhenUnconnected=off
  vel_K_O_mDs : Outport  Port=5  PortDimensions=[3,1]  VectorParamsAs1DForOutWhenUnconnected=off
  longlat : Outport  Port=6  PortDimensions=[2,1]  VectorParamsAs1DForOutWhenUnconnected=off
  pos_O : Outport  Port=7  PortDimensions=[3,1]  VectorParamsAs1DForOutWhenUnconnected=off
  Va : Outport  Port=8  PortDimensions=1  VectorParamsAs1DForOutWhenUnconnected=off
  eta_a : Outport  Port=9  PortDimensions=[3,1]  VectorParamsAs1DForOutWhenUnconnected=off
  EULER : Outport  Port=10  PortDimensions=[3,1]  VectorParamsAs1DForOutWhenUnconnected=off
  mu_k : Outport  Port=11  PortDimensions=1  VectorParamsAs1DForOutWhenUnconnected=off
  a_B : Outport  Port=12  PortDimensions=[3,1]  VectorParamsAs1DForOutWhenUnconnected=off
  pos_W : Outport  Port=13  PortDimensions=[3,1]  VectorParamsAs1DForOutWhenUnconnected=off
  vel_W : Outport  Port=14  PortDimensions=[3,1]  VectorParamsAs1DForOutWhenUnconnected=off
  M_OB : Outport  Port=15  PortDimensions=[3,3]  VectorParamsAs1DForOutWhenUnconnected=off
  tag scope: chi_a_dot_real=global, gamma_a_dot_real=global
  wires:
  Delay5/1 -> pathangles_a/1
  Delay4/1 -> M_OB/1, Estimations/6(M_OB)
  Torques_B/1 -> MATLAB Function2/5(Torques_B)
  MATLAB Function2/2(M_OB) -> Delay4/1
  F_a_B/1 -> MATLAB Function2/2(F_a_B), Delay/1
  Mux/1 -> Delay14/1
  MATLAB Function2/3(omega_OB_B_dot) -> Integrator5/1
  MATLAB Function2/4(longlat_dot) -> Integrator6/1, Selector/1, Selector1/1
  MATLAB Function2/1(vel_K_B_dot) -> Delay11/1, Integrator1/1
  v_w_W/1 -> Estimations/5(v_w_W)
  Integrator1/1 -> Estimations/4(v_k_B), MATLAB Function2/1(v_k_B), v_k_B/1
  F_p_B/1 -> MATLAB Function2/3(F_p_B), Delay1/1
  Estimations/8(pathangles_a) -> Delay5/1
  Estimations/9(pathangles_k) -> Delay9/1
  Estimations/2(Va) -> Delay7/1
  Delay7/1 -> Va/1
  Estimations/3(mu_a) -> Mux/1
  Delay2/1 -> [chi_a_dot_real]
  Estimations/6(chi_a_dot_real) -> Delay2/1
  Estimations/7(gamma_a_dot_real) -> Delay3/1
  Delay3/1 -> [gamma_a_dot_real]
  MATLAB Function2/5(eta_EULER_dot) -> Integrator/1
  Integrator/1 -> MATLAB Function2/9(EULER), Estimations/8(EULER), EULER/1
  Integrator5/1 -> MATLAB Function2/7(omega_OB_B), omega_OB_B/1
  Estimations/1(mu_k) -> Delay13/1
  Integrator6/1 -> MATLAB Function2/8(longlat), Estimations/7(longlat), longlat/1
  Delay13/1 -> mu_k/1
  Delay14/1 -> eta_a/1
  Delay9/1 -> pathangles_k/1
  Estimations/4(alpha) -> Mux/2
  Estimations/5(beta) -> Mux/3
  F_t_W/1 -> MATLAB Function2/4(F_t_W), Dot Product/1, Dot Product/2
  Dot Product/1 -> Sqrt/1
  Delay11/1 -> a_B/1
  MATLAB Function2/6(h_tau_dot) -> Integrator2/1
  Integrator2/1 -> MATLAB Function2/10(h_tau), Estimations/9(h_tau)
  Estimations/12(pos_O) -> pos_O/1
  Estimations/13(v_k_W) -> MATLAB Function2/6(vel_k_W), vel_W/1
  Estimations/11(pos_W) -> pos_W/1
  Estimations/10(v_k_O) -> vel_K_O_mDs/1
  Delay/1 -> Estimations/2(F_a_B)
  Delay1/1 -> Estimations/3(F_p_B)
  Sqrt/1 -> Estimations/1(Ft)
  Selector/1 -> Goto/1
  Selector1/1 -> Goto1/1

== system Dyn_6DoF_v2_0_r2019b/AirborneSystem/FlightControlSystem/AttitudeAndRateLoop ==
  mu_a_cmd : Inport
  M_a_B_est : Inport  Port=2
  flightMode : Inport  Port=3
  alpha_a_cmd : Inport  Port=4
  StateEstimation_Bus : Inport  Port=5
  AttitudeController : Subsystem
  Compare To Constant : simulink/Logic and Bit Operations/Compare To Constant  relop===  const=6  OutDataTypeStr=boolean
  RateLoop : Subsystem
  u_rb : Outport  VectorParamsAs1DForOutWhenUnconnected=off
  wires:
  M_a_B_est/1 -> RateLoop/3(M_a_B_est)
  RateLoop/1(u_rb) -> u_rb/1
  mu_a_cmd/1 -> AttitudeController/2(mu_a_cmd)
  AttitudeController/1(omega_OB_B_cmd) -> RateLoop/2(omega_OB_B_cmd)
  alpha_a_cmd/1 -> AttitudeController/3(alpha_a_cmd)
  StateEstimation_Bus/1 -> RateLoop/1(StateEstimation_Bus), AttitudeController/1(StateEstimation_Bus)
  flightMode/1 -> Compare To Constant/1
  Compare To Constant/1 -> AttitudeController/4(reset)

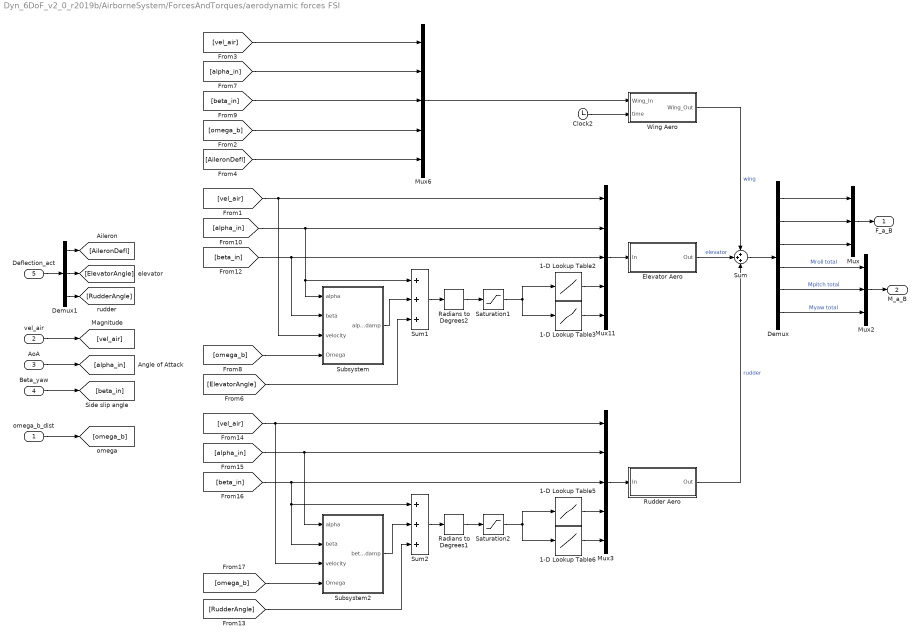
== system Dyn_6DoF_v2_0_r2019b/AirborneSystem/ForcesAndTorques/aerodynamic forces FSI ==
  omega_b_dist : Inport
  vel_air : Inport  Port=2
  AoA : Inport  Port=3
  Beta_yaw : Inport  Port=4
  Deflection_act : Inport  Port=5
  1-D Lookup Table2 : Lookup_n-D  NumberOfTableDimensions=1  BreakpointsForDimension1=DE2019.alpha  BreakpointsForDimension2=[1 1]  Table=DE2019.el_cL'  InternalRulePriority=Speed  RndMeth=Simplest  InputSameDT=on
  1-D Lookup Table3 : Lookup_n-D  NumberOfTableDimensions=1  BreakpointsForDimension1=DE2019.alpha  BreakpointsForDimension2=[1 1]  Table=DE2019.el_cD'  InternalRulePriority=Speed  RndMeth=Simplest  InputSameDT=on
  1-D Lookup Table5 : Lookup_n-D  NumberOfTableDimensions=1  BreakpointsForDimension1=DE2019.alpha  BreakpointsForDimension2=[1 1]  Table=DE2019.vs_cL'  InternalRulePriority=Speed  RndMeth=Simplest  InputSameDT=on
  1-D Lookup Table6 : Lookup_n-D  NumberOfTableDimensions=1  BreakpointsForDimension1=DE2019.alpha  BreakpointsForDimension2=[1 1]  Table=DE2019.vs_cD'  InternalRulePriority=Speed  RndMeth=Simplest  InputSameDT=on
  Clock2 : Clock
  Demux : Demux  Outputs=6
  Demux1 : Demux  Outputs=3
  Elevator Aero : Subsystem
  Mux : Mux  Inputs=3
  Mux11 : Mux  Inputs=5
  Mux2 : Mux  Inputs=3
  Mux3 : Mux  Inputs=5
  Mux6 : Mux  Inputs=5
  Radians to Degrees1 : simulink_extras/Transformations/Radians to Degrees
  Radians to Degrees2 : simulink_extras/Transformations/Radians to Degrees
  Rudder Aero : Subsystem
  Saturation1 : Saturate  UpperLimit=max(DE2019.alpha)  LowerLimit=min(DE2019.alpha)
  Saturation2 : Saturate  UpperLimit=max(DE2019.alpha)  LowerLimit=min(DE2019.alpha)
  Subsystem : Subsystem
  Subsystem2 : Subsystem
  Sum : Sum  Inputs=+++
  Sum1 : Sum  Inputs=+++
  Sum2 : Sum  Inputs=+++
  Wing Aero : Subsystem  TreatAsAtomicUnit=on  SystemSampleTime=0.01
  F_a_B : Outport  VectorParamsAs1DForOutWhenUnconnected=off
  M_a_B : Outport  Port=2  VectorParamsAs1DForOutWhenUnconnected=off
  wires:
  Sum/1 -> Demux/1
  Mux6/1 -> Wing Aero/1(Wing_In)
  omega_b_dist/1 -> [omega_b]
  Demux1/2 -> [ElevatorAngle]
  vel_air/1 -> [vel_air]
  [vel_air] -> Subsystem/3(velocity), Mux11/1
  Clock2/1 -> Wing Aero/2(time)
  Elevator Aero/1(Out) -> Sum/2  "elevator"
  Wing Aero/1(Wing_Out) -> Sum/1  "wing"
  Deflection_act/1 -> Demux1/1
  Demux1/1 -> [AileronDefl]
  Demux1/3 -> [RudderAngle]
  AoA/1 -> [alpha_in]
  Beta_yaw/1 -> [beta_in]
  [ElevatorAngle] -> Sum1/3
  [omega_b] -> Subsystem/4(Omega)
  [alpha_in] -> Subsystem/1(alpha), Sum1/1, Mux11/2
  [beta_in] -> Subsystem/2(beta), Mux11/3
  Demux/1 -> Mux/1
  Demux/2 -> Mux/2
  Demux/3 -> Mux/3
  Mux/1 -> F_a_B/1
  Demux/6 -> Mux2/3  "Myaw total"
  Mux2/1 -> M_a_B/1
  Demux/4 -> Mux2/1  "Mroll total"
  Demux/5 -> Mux2/2  "Mpitch total"
  Sum1/1 -> Radians to Degrees2/1
  Radians to Degrees2/1 -> Saturation1/1
  Saturation1/1 -> 1-D Lookup Table2/1, 1-D Lookup Table3/1
  Subsystem/1(alpha_damp) -> Sum1/2
  1-D Lookup Table2/1 -> Mux11/4
  1-D Lookup Table3/1 -> Mux11/5
  Mux11/1 -> Elevator Aero/1(In)
  Radians to Degrees1/1 -> Saturation2/1
  [alpha_in] -> Subsystem2/1(alpha), Mux3/2
  [beta_in] -> Subsystem2/2(beta), Sum2/1, Mux3/3
  [RudderAngle] -> Sum2/3
  [omega_b] -> Subsystem2/4(Omega)
  Saturation2/1 -> 1-D Lookup Table6/1, 1-D Lookup Table5/1
  [vel_air] -> Subsystem2/3(velocity), Mux3/1
  Subsystem2/1(beta_damp) -> Sum2/2
  1-D Lookup Table6/1 -> Mux3/5
  1-D Lookup Table5/1 -> Mux3/4
  Sum2/1 -> Radians to Degrees1/1
  Mux3/1 -> Rudder Aero/1(In)
  Rudder Aero/1(Out) -> Sum/3  "rudder"
  [vel_air] -> Mux6/1
  [alpha_in] -> Mux6/2
  [beta_in] -> Mux6/3
  [omega_b] -> Mux6/4
  [AileronDefl] -> Mux6/5

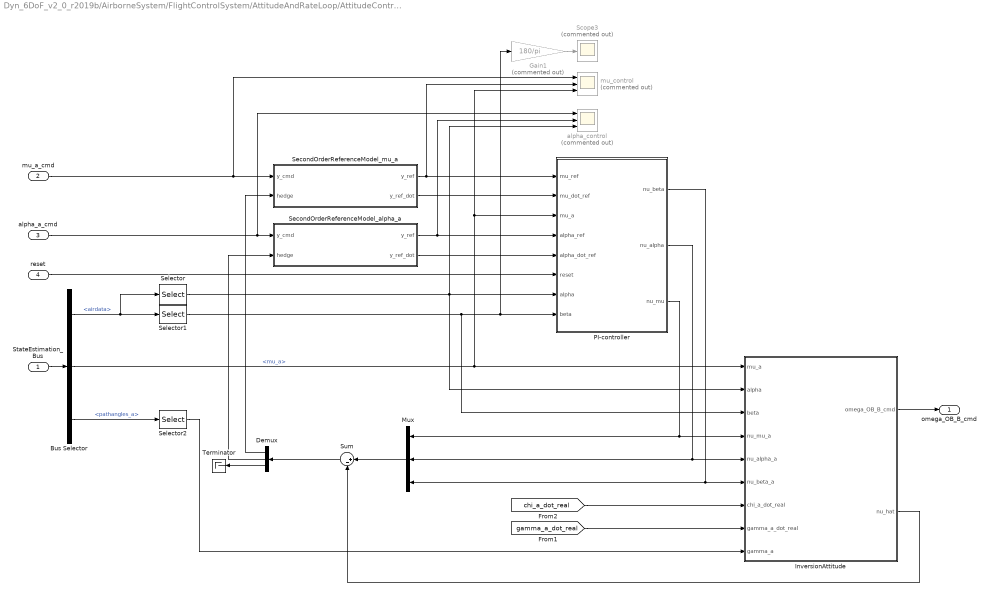
== system Dyn_6DoF_v2_0_r2019b/AirborneSystem/FlightControlSystem/AttitudeAndRateLoop/AttitudeController ==
  StateEstimation_Bus : Inport
  mu_a_cmd : Inport  Port=2
  alpha_a_cmd : Inport  Port=3
  reset : Inport  Port=4
  Bus Selector : BusSelector  OutputSignals=airdata,mu_a,pathangles_a
  Demux : Demux  Outputs=3
  Gain1 : Gain  Commented=on  Gain=180/pi
  InversionAttitude : MATLAB Function  TreatAsAtomicUnit=on
  Mux : Mux  Inputs=3
  PI-controller : Subsystem  mask{Kp_mu=params.Kp_mu, Kp_alpha=params.Kp_alpha, Kp_beta=params.Kp_beta, Ki_mu=params.Ki_mu, Ki_alpha=params.Ki_alpha, Ki_beta=params.Ki_beta}
  Scope3 : Scope  Commented=on
  SecondOrderReferenceModel_alpha_a : Subsystem  mask{omega0_max=params.w0_alpha, zeta0=1, y_max=constr.alpha_a_max, y_min=constr.alpha_a_min, yd_max=inf, yd_min=-inf, y2d_max=inf, y2d_min=-inf}
  SecondOrderReferenceModel_mu_a : Subsystem  mask{omega0_max=params.w0_mu, zeta0=1, y_max=constr.mu_a_max, y_min=constr.mu_a_min, yd_max=inf, yd_min=-inf, y2d_max=inf, y2d_min=-inf}
  Selector : Selector  InputPortWidth=3  IndexOptions=Index vector (dialog)  Indices=2  OutputSizes=1
  Selector1 : Selector  InputPortWidth=3  IndexOptions=Index vector (dialog)  Indices=3  OutputSizes=1
  Selector2 : Selector  InputPortWidth=2  IndexOptions=Index vector (dialog)  Indices=2  OutputSizes=1
  Sum : Sum  Inputs=|+-
  Terminator : Terminator
  alpha_control : Scope  Commented=on  NumInputPorts=3
  mu_control : Scope  Commented=on  NumInputPorts=3
  omega_OB_B_cmd : Outport  PortDimensions=[3,1]  VectorParamsAs1DForOutWhenUnconnected=off
  wires:
  Demux/2 -> SecondOrderReferenceModel_alpha_a/2(hedge)
  Demux/1 -> SecondOrderReferenceModel_mu_a/2(hedge)
  Sum/1 -> Demux/1
  InversionAttitude/2(nu_hat) -> Sum/2
  Mux/1 -> Sum/1
  mu_a_cmd/1 -> mu_control/1, SecondOrderReferenceModel_mu_a/1(y_cmd)
  alpha_a_cmd/1 -> alpha_control/1, SecondOrderReferenceModel_alpha_a/1(y_cmd)
  Selector2/1 -> InversionAttitude/9(gamma_a)
  Bus Selector/3 -> Selector2/1  "<pathangles_a>"
  Bus Selector/2 -> mu_control/3, PI-controller/3(mu_a), InversionAttitude/1(mu_a)  "<mu_a>"
  Bus Selector/1 -> Selector/1, Selector1/1  "<airdata>"
  StateEstimation_Bus/1 -> Bus Selector/1
  [gamma_a_dot_real] -> InversionAttitude/8(gamma_a_dot_real)
  [chi_a_dot_real] -> InversionAttitude/7(chi_a_dot_real)
  InversionAttitude/1(omega_OB_B_cmd) -> omega_OB_B_cmd/1
  PI-controller/1(nu_beta) -> InversionAttitude/6(nu_beta_a), Mux/3
  PI-controller/3(nu_mu) -> InversionAttitude/4(nu_mu_a), Mux/1
  SecondOrderReferenceModel_mu_a/1(y_ref) -> PI-controller/1(mu_ref), mu_control/2
  SecondOrderReferenceModel_mu_a/2(y_ref_dot) -> PI-controller/2(mu_dot_ref)
  SecondOrderReferenceModel_alpha_a/1(y_ref) -> alpha_control/2, PI-controller/4(alpha_ref)
  SecondOrderReferenceModel_alpha_a/2(y_ref_dot) -> PI-controller/5(alpha_dot_ref)
  PI-controller/2(nu_alpha) -> InversionAttitude/5(nu_alpha_a), Mux/2
  reset/1 -> PI-controller/6(reset)
  Demux/3 -> Terminator/1
  Selector/1 -> InversionAttitude/2(alpha), PI-controller/7(alpha), alpha_control/3
  Selector1/1 -> InversionAttitude/3(beta), Gain1/1, PI-controller/8(beta)
  Gain1/1 -> Scope3/1

== system Dyn_6DoF_v2_0_r2019b/AirborneSystem/FlightControlSystem/AttitudeAndRateLoop/RateLoop ==
  StateEstimation_Bus : Inport
  omega_OB_B_cmd : Inport  Port=2
  M_a_B_est : Inport  Port=3
  "Actuatormodel " : Subsystem  ReferencedSubsystem=Actuatormodel_R2019B
  Bus Selector : BusSelector  OutputSignals=airdata,omega_OB_B
  ControlAllocation : Subsystem
  Rate_Loop : Subsystem
  u_rb : Outport  VectorParamsAs1DForOutWhenUnconnected=off
  wires:
  Bus Selector/2 -> Rate_Loop/1(omega_OB_B)  "<omega_OB_B>"
  omega_OB_B_cmd/1 -> Rate_Loop/2(omega_OB_B_cmd)
  StateEstimation_Bus/1 -> Bus Selector/1
  Rate_Loop/1(delta_M_cmd) -> ControlAllocation/3(Delta_mom_cmd)
  M_a_B_est/1 -> Rate_Loop/3(M_a_B_est)
  Bus Selector/1 -> ControlAllocation/2(airdata)  "<airdata>"
  "Actuatormodel "/1 -> ControlAllocation/1(deflections_actuator_output)
  ControlAllocation/1(deflections_cmd) -> u_rb/1, "Actuatormodel "/1

== system Dyn_6DoF_v2_0_r2019b/AirborneSystem/ForcesAndTorques/aerodynamic forces FSI/Elevator Aero ==
  In : Inport
  Elevator_aero : MATLAB Function  TreatAsAtomicUnit=on
  Out : Outport  VectorParamsAs1DForOutWhenUnconnected=off
  wires:
  Elevator_aero/1(out) -> Out/1
  In/1 -> Elevator_aero/1(input)

== system Dyn_6DoF_v2_0_r2019b/AirborneSystem/ForcesAndTorques/aerodynamic forces FSI/Rudder Aero ==
  In : Inport
  Rudder_aero : MATLAB Function  TreatAsAtomicUnit=on
  Out : Outport  VectorParamsAs1DForOutWhenUnconnected=off
  wires:
  Rudder_aero/1(out) -> Out/1
  In/1 -> Rudder_aero/1(input)

== system Dyn_6DoF_v2_0_r2019b/AirborneSystem/ForcesAndTorques/aerodynamic forces FSI/Subsystem ==
  alpha : Inport
  beta : Inport  Port=2
  velocity : Inport  Port=3
  Omega : Inport  Port=4
  Atan2 : Trigonometry  Operator=atan2
  Constant : Constant  Value=(DE2019.x_el+DE2019.c_el*0.25)
  Cos : Trigonometry  Operator=cos
  Cos1 : Trigonometry  Operator=cos
  Product : Product  Inputs=3
  Product1 : Product  Commented=on
  Product2 : Product  Commented=on  Inputs=3
  Product3 : Product
  Selector : Selector  InputPortWidth=3  IndexOptions=Index vector (dialog)  Indices=1  OutputSizes=1
  Sin : Trigonometry  Commented=on
  Sin1 : Trigonometry  Commented=on
  Terminator : Terminator  Commented=on
  Terminator1 : Terminator  Commented=on
  alpha_damp : Outport  VectorParamsAs1DForOutWhenUnconnected=off
  wires:
  alpha/1 -> Sin/1, Cos/1
  beta/1 -> Sin1/1, Cos1/1
  Product/1 -> Atan2/2
  Product1/1 -> Terminator/1
  Product2/1 -> Terminator1/1
  velocity/1 -> Product1/1, Product2/1, Product/1
  Cos/1 -> Product/2
  Cos1/1 -> Product2/3, Product/3
  Sin1/1 -> Product1/2
  Sin/1 -> Product2/2
  Constant/1 -> Product3/1
  Omega/1 -> Selector/1
  Selector/1 -> Product3/2
  Product3/1 -> Atan2/1
  Atan2/1 -> alpha_damp/1

== system Dyn_6DoF_v2_0_r2019b/AirborneSystem/ForcesAndTorques/aerodynamic forces FSI/Subsystem2 ==
  alpha : Inport
  beta : Inport  Port=2
  velocity : Inport  Port=3
  Omega : Inport  Port=4
  Atan2 : Trigonometry  Operator=atan2
  Constant : Constant  Value=(DE2019.x_el+DE2019.c_el*0.25)
  Cos : Trigonometry  Operator=cos
  Cos1 : Trigonometry  Operator=cos
  Gain : Gain  Gain=-1
  Product : Product  Inputs=3
  Product1 : Product  Commented=on
  Product2 : Product  Commented=on  Inputs=3
  Product3 : Product
  Selector : Selector  InputPortWidth=3  IndexOptions=Index vector (dialog)  Indices=3  OutputSizes=1
  Sin : Trigonometry  Commented=on
  Sin1 : Trigonometry  Commented=on
  beta_damp : Outport  VectorParamsAs1DForOutWhenUnconnected=off
  wires:
  Atan2/1 -> Gain/1
  Gain/1 -> beta_damp/1
  Product3/1 -> Atan2/1
  Sin1/1 -> Product1/2
  alpha/1 -> Sin/1, Cos/1
  Cos/1 -> Product/2
  Omega/1 -> Selector/1
  Sin/1 -> Product2/2
  Product1/1 -> ?
  Constant/1 -> Product3/1
  velocity/1 -> Product1/1, Product2/1, Product/1
  Product2/1 -> ?
  beta/1 -> Sin1/1, Cos1/1
  Product/1 -> Atan2/2
  Cos1/1 -> Product2/3, Product/3
  Selector/1 -> Product3/2

== system Dyn_6DoF_v2_0_r2019b/AirborneSystem/ForcesAndTorques/aerodynamic forces FSI/Wing Aero ==
  Wing_In : Inport
  time : Inport  Port=2
  Constant : Constant
  Constant1 : Constant  Value=0
  If : If  IfExpression=u1 >= 1
  If Action Subsystem : Subsystem  TreatAsAtomicUnit=on
  If Action Subsystem1 : Subsystem  TreatAsAtomicUnit=on
  Merge : Merge
  Switch : Switch  Threshold=simInit.FSI_switchtime
  Wing_Out : Outport  VectorParamsAs1DForOutWhenUnconnected=off
  wires:
  If/1 -> If Action Subsystem/Action
  If/2 -> If Action Subsystem1/Action
  If Action Subsystem1/1(Simple_out) -> Merge/2
  If Action Subsystem/1(FSI_out) -> Merge/1
  Merge/1 -> Wing_Out/1
  time/1 -> Switch/2, If Action Subsystem/2(simTime)
  Constant/1 -> Switch/1
  Constant1/1 -> Switch/3
  Switch/1 -> If/1
  Wing_In/1 -> If Action Subsystem1/1(Simple_in), If Action Subsystem/1(FSI_in)
